simulink model "TRAS_LQI"  (R2021b)
settings: Solver=ode5  StartTime=0.0  StopTime=999  FixedStep=0.01  RelTol=1e-3  AbsTol=1e-6
values from neighbouring files (symbols this model uses):
  D = params.D    [x00_pendulum_identification.m]
  K = [9.60215440973 2.43688595265 0.00134146532326 3.16227766017]    [LQI_SETPOINT_CHANGE.mat]    (also in LQI_losowe_zaklocenie_i_maksymalne_zaklocenie_kilka_razy(ost_naj).mat; LQI_sam_z_ciezarem_znowu_sam.mat; LQR_losowe_zaklocenie_i_maksymalne_zaklocenie.mat = [8.82696664421 2.33839377811 0.00131075429192]; LQR_sam_z_ciezarem_znowu_sam.mat = [8.82696664421 2.33839377811 0.00131075429192])
  u_ref = u_ref_sol    [x03_pitch_control_model.m]
  x_ref = [theta_p_setpoint; 1e-12; omega_ref_sol]    [x03_pitch_control_model.m]
libraries: simulink x4, dspstat3 x3
settings Model: SimulationMode=external  ExtModeTrigDuration=12000  ExtModeTrigLevel=0.400000  Creator=jims  LastModifiedBy=STUDENT
settings SolverCC: AutoScaleAbsTol=off  AlgebraicLoopSolver=TrustRegion
settings DataIOCC: ExternalInput=[]  InitialState=[]  MaxDataPoints=5000  SaveFormat=Array  SignalLoggingSaveFormat=ModelDataLogs  SaveOutput=off  SaveTime=off  ReturnWorkspaceOutputs=off  SignalLoggingName=sigsOut
settings OptimizationCC: BooleanDataType=off  ExpressionDepthLimit=2147483647  InitFltsAndDblsToZero=on  LifeSpan=inf
settings DebuggingCC: SaveWithParameterizedLinksMsg=none  MultiTaskDSMMsg=warning  MultiTaskCondExecSysMsg=none  IntegerOverflowMsg=none  StateNameClashWarn=warning  SFUnexpectedBacktrackingDiag=warning  SFNoUnconditionalDefaultTransitionDiag=warning  SFExecutionAtInitializationDiag=none  SFMachineParentedDataDiag=warning  IntegerSaturationMsg=none  ArithmeticOperatorsInVariantConditions=warning
settings HardwareCC: TargetBitPerLong=64  TargetBitPerPointer=64  TargetIntDivRoundTo=Zero  TargetEndianess=LittleEndian  TargetWordSize=64  TargetHWDeviceType=Intel->x86-64
settings ModelReferenceCC: PropagateSignalLabelsOutOfModel=off
settings SFSimCC: SimUseLocalCustomCode=off  CustomCodeUndefinedFunction=UseInterfaceOnly
settings RTWCC: Description=Simulink Desktop Real-Time  SystemTargetFile=sldrt.tlc  TemplateMakefile=sldrt.tmf  RTWUseLocalCustomCode=off  RTWCompilerOptimization=on
settings CodeAppCC: MaxIdLength=95  StateflowObjectComments=on
settings SimulinkDesktopRealTimeCC: TargetFcnLib=ansi_tfl_tmw.mat  TargetPreCompLibLocation=C:\apps\MATLAB\R2021b\toolbox\sldrt\lib\win64  TargetLangStandard=C89/C90 (ANSI)  ModelReferenceCompliant=off  CompOptLevelCompliant=off  SupportVariableSizeSignals=off
settings ConfigComp: CovMetricSettings=dw  CovSaveCumulativeToWorkspaceVar=on  CovSaveSingleToWorkspaceVar=on  CovExternalEMLEnable=off

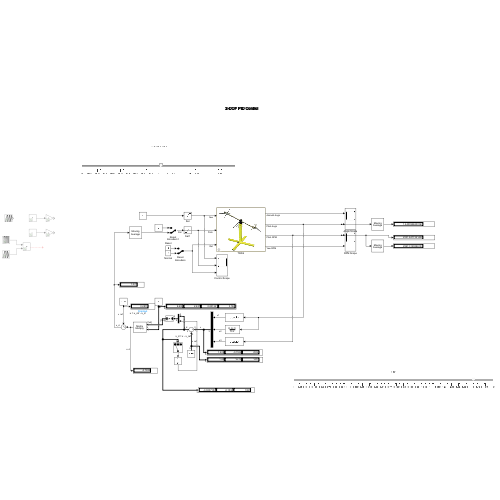
[thumbnail: Simulink's stored preview of the top-level diagram]
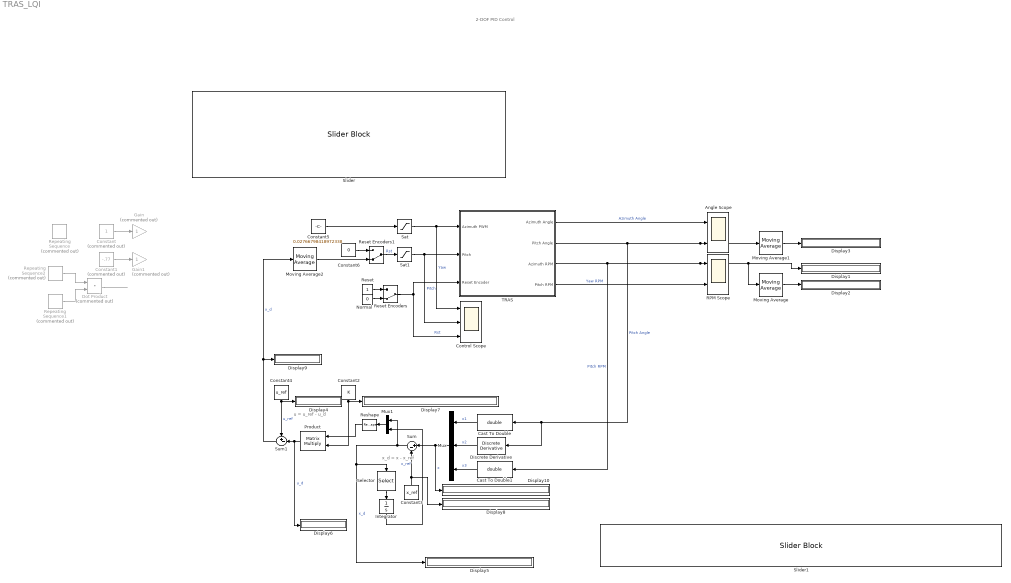
== system TRAS_LQI ==
  note: x_d = x - x_ref
  note: 2-DOF PID Control
  note: u = u_ref - u_d
  Angle Scope : Scope  NumInputPorts=2
  Cast To Double : DataTypeConversion  OutDataTypeStr=double
  Cast To Double1 : DataTypeConversion  OutDataTypeStr=double
  Constant : Constant  Commented=on
  Constant1 : Constant  Commented=on  Value=-.77
  Constant2 : Constant  Value=K
  Constant3 : Constant  Value=x_ref
  Constant4 : Constant  Value=u_ref
  Constant5 : Constant  Value=0.02766798418972338
  Constant6 : Constant  Value=0
  Control Scope : Scope  NumInputPorts=3
  Discrete Derivative : simulink/Discrete/Discrete Derivative  gainval=1.0  ICPrevScaledInput=0.0  OutMin=[]  OutMax=[]  OutDataType=fixdt(1, 16)  OutScaling=2^-10  DoSatur=off
  Display{1..10} (10 alike) : Display
  Dot Product : DotProduct  Commented=on  InputSameDT=on  OutDataTypeStr=Inherit: Inherit via internal rule
  Gain : Gain  Commented=on
  Gain1 : Gain  Commented=on
  Integrator : Integrator
  Moving Average : dspstat3/Moving Average  Method=Sliding window  ForgettingFactorPort=off  SpecifyWindowLength=on  WindowLength=100  ForgettingFactor=0.9  SimulateUsing=Code generation
  Moving Average1 : dspstat3/Moving Average  Method=Sliding window  ForgettingFactorPort=off  SpecifyWindowLength=on  WindowLength=100  ForgettingFactor=0.9  SimulateUsing=Code generation
  Moving Average2 : dspstat3/Moving Average  Method=Sliding window  ForgettingFactorPort=off  SpecifyWindowLength=on  WindowLength=10  ForgettingFactor=0.9  SimulateUsing=Code generation
  Mux : Mux  Inputs=3
  Mux1 : Mux  Inputs=2
  Normal : Constant  Value=0
  Product : Product  Multiplication=Matrix(*)
  RPM Scope : Scope  NumInputPorts=2
  Repeating Sequence : simulink/Sources/Repeating Sequence  Commented=on  rep_seq_t=[0 1 1.001 2 2.001 3 3.001 4 4.001 5 5.001 6 6.001 7 7.001 8 8.001 9 9.001 10 10.001 11]*10.  rep_seq_y=[0 0 1 1 2 2 3 3 4 4 5 5 6 6 7 7 8 8 9 9 10 10]/10
  Repeating Sequence1 : simulink/Sources/Repeating Sequence  Commented=on  rep_seq_t=[0 1 1.001 2 2.001 3 3.001 4 4.001 5 5.001 6 6.001 7 7.001 8 8.001 9 9.001 10 10.001 11]*20  rep_seq_y=[0 0 1 1 2 2 3 3 4 4 5 5 6 6 7 7 8 8 9 9 10 10]/10
  Repeating Sequence2 : simulink/Sources/Repeating Sequence  Commented=on  rep_seq_t=[0 10 10.001 20]  rep_seq_y=[0 0 1 1]
  Reset : Constant
  Reset Encoders : ManualSwitch  CurrentSetting=0
  Reset Encoders1 : ManualSwitch  CurrentSetting=0
  Reshape : Reshape  OutputDimensionality=Row vector (2-D)
  Sat : Saturate  UpperLimit=1  LowerLimit=-1
  Sat1 : Saturate  UpperLimit=1  LowerLimit=-1
  Selector : Selector  InputPortWidth=3  IndexOptions=Index vector (dialog)  Indices=[1]  OutputSizes=1
  Slider : SliderBlock  ScaleMin=-1  ScaleMax=1
  Slider1 : SliderBlock  ScaleMax=1.6
  Sum : Sum  Inputs=|+-
  Sum1 : Sum  Inputs=+-|
  TRAS : Subsystem  mask{BaseAddress=57088, T0=0.01}
      mask prompts: BaseAddress "Base Address:"; T0 "Sampling Period:"
      mask Display: image('TRAS.JPG')
  wires:
  Sat/1 -> TRAS/1(Azimuth PWM), Control Scope/1  "Yaw"
  Sat1/1 -> Control Scope/2, TRAS/2(Pitch)  "Pitch"
  Reset Encoders/1 -> TRAS/3(Reset Encoder), Control Scope/3  "Rst"
  Reset/1 -> Reset Encoders/1
  Normal/1 -> Reset Encoders/2
  TRAS/4(Pitch RPM) -> RPM Scope/2  "Yaw RPM"
  TRAS/3(Azimuth RPM) -> Cast To Double1/1, Display1/1, Moving Average/1, RPM Scope/1  "Pitch RPM"
  TRAS/1(Azimuth Angle) -> Angle Scope/1  "Azimuth Angle"
  TRAS/2(Pitch Angle) -> Discrete Derivative/1, Cast To Double/1, Moving Average1/1, Angle Scope/2  "Pitch Angle"
  Moving Average/1 -> Display2/1
  Moving Average1/1 -> Display3/1
  Repeating Sequence2/1 -> Dot Product/1
  Repeating Sequence1/1 -> Dot Product/2
  Constant1/1 -> Gain1/1
  Dot Product/1 -> ?
  Constant/1 -> Gain/1
  Cast To Double/1 -> Mux/1  "x1"
  Cast To Double1/1 -> Mux/3  "x3"
  Discrete Derivative/1 -> Mux/2  "x2"
  Mux/1 -> Display10/1, Sum/1  "x"
  Constant3/1 -> Display8/1, Sum/2  "x_ref"
  Sum/1 -> Selector/1, Display5/1, Mux1/1  "x_d"
  Product/1 -> Display6/1, Sum1/2  "u_d"
  Constant4/1 -> Display4/1, Sum1/1  "u_ref"
  Sum1/1 -> Display9/1, Moving Average2/1  "x_d"
  Constant2/1 -> Product/2, Display7/1
  Reset Encoders1/1 -> Sat1/1  "Rst"
  Constant6/1 -> Reset Encoders1/1
  Moving Average2/1 -> Reset Encoders1/2
  Selector/1 -> Integrator/1
  Integrator/1 -> Mux1/2
  Mux1/1 -> Reshape/1
  Reshape/1 -> Product/1
  Constant5/1 -> Sat/1

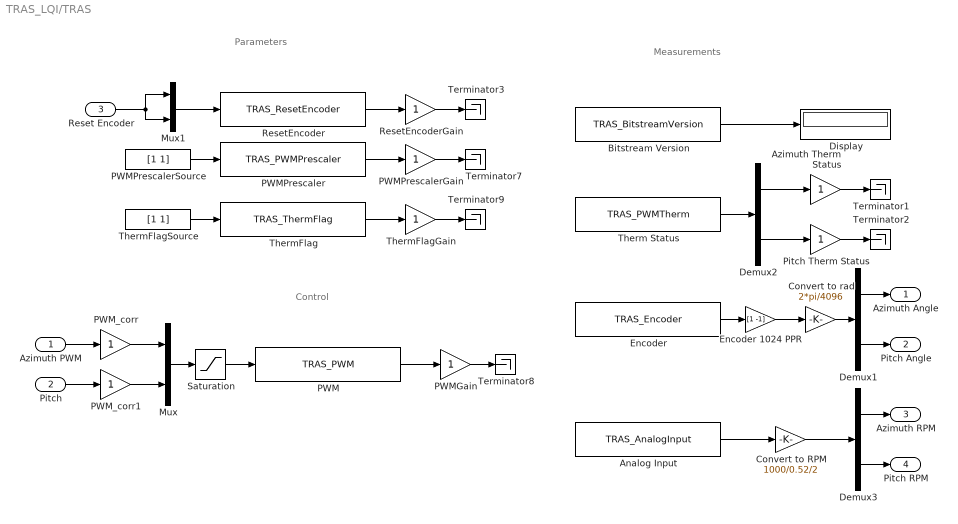
== system TRAS_LQI/TRAS ==
  note: Parameters
  note: Control
  note: Measurements
  Azimuth PWM : Inport
  Pitch : Inport  Port=2
  Reset Encoder : Inport  Port=3
  Analog Input : S-Function  FunctionName=TRAS_AnalogInput  Parameters=BaseAddress, [1 0], [1 1], T0  SFunctionDeploymentMode=off  EnableBusSupport=off
  Azimuth Therm Status : Gain  SaturateOnIntegerOverflow=on  OutDataTypeStr=Inherit: Same as input  ParamDataTypeStr=Inherit: Same as input
  Bitstream Version : S-Function  FunctionName=TRAS_BitstreamVersion  Parameters=BaseAddress, T0  SFunctionDeploymentMode=off  EnableBusSupport=off
  Convert to RPM : Gain  Gain=1000/0.52/2  SaturateOnIntegerOverflow=on  OutDataTypeStr=Inherit: Same as input  ParamDataTypeStr=Inherit: Same as input
  Convert to rad : Gain  Gain=2*pi/4096  SaturateOnIntegerOverflow=on  OutDataTypeStr=Inherit: Same as input  ParamDataTypeStr=Inherit: Same as input
  Demux1 : Demux  Outputs=2
      settings: DisplayOption=none
  Demux2 : Demux  Outputs=2
      settings: DisplayOption=none
  Demux3 : Demux  Outputs=2
      settings: DisplayOption=none
  Display : Display
  Encoder : S-Function  FunctionName=TRAS_Encoder  Parameters=BaseAddress, T0  SFunctionDeploymentMode=off  EnableBusSupport=off
  Encoder 1024 PPR : Gain  Gain=[1 -1]  SaturateOnIntegerOverflow=on  OutDataTypeStr=Inherit: Same as input  ParamDataTypeStr=Inherit: Same as input
  Mux : Mux  Inputs=2
  Mux1 : Mux  Inputs=2
  PWM : S-Function  FunctionName=TRAS_PWM  Parameters=BaseAddress, T0  SFunctionDeploymentMode=off  EnableBusSupport=off
  PWMGain : Gain  SaturateOnIntegerOverflow=on  OutDataTypeStr=Inherit: Same as input  ParamDataTypeStr=Inherit: Same as input
  PWMPrescaler : S-Function  FunctionName=TRAS_PWMPrescaler  Parameters=BaseAddress, T0  SFunctionDeploymentMode=off  EnableBusSupport=off
  PWMPrescalerGain : Gain  SaturateOnIntegerOverflow=on  OutDataTypeStr=Inherit: Same as input  ParamDataTypeStr=Inherit: Same as input
  PWMPrescalerSource : Constant  Value=[1 1]
  PWM_corr : Gain  SaturateOnIntegerOverflow=on  OutDataTypeStr=Inherit: Same as input  ParamDataTypeStr=Inherit: Same as input
  PWM_corr1 : Gain  SaturateOnIntegerOverflow=on  OutDataTypeStr=Inherit: Same as input  ParamDataTypeStr=Inherit: Same as input
  Pitch Therm Status : Gain  SaturateOnIntegerOverflow=on  OutDataTypeStr=Inherit: Same as input  ParamDataTypeStr=Inherit: Same as input
  ResetEncoder : S-Function  FunctionName=TRAS_ResetEncoder  Parameters=BaseAddress, T0  SFunctionDeploymentMode=off  EnableBusSupport=off
  ResetEncoderGain : Gain  SaturateOnIntegerOverflow=on  OutDataTypeStr=Inherit: Same as input  ParamDataTypeStr=Inherit: Same as input
  Saturation : Saturate  UpperLimit=1  LowerLimit=-1
  Terminator{1..3,7..9} (6 alike) : Terminator
  Therm Status : S-Function  FunctionName=TRAS_PWMTherm  Parameters=BaseAddress, T0  SFunctionDeploymentMode=off  EnableBusSupport=off
  "ThermFlag " : S-Function  FunctionName=TRAS_ThermFlag  Parameters=BaseAddress, T0  SFunctionDeploymentMode=off  EnableBusSupport=off
  ThermFlagGain : Gain  SaturateOnIntegerOverflow=on  OutDataTypeStr=Inherit: Same as input  ParamDataTypeStr=Inherit: Same as input
  ThermFlagSource : Constant  Value=[1 1]
  Azimuth Angle : Outport
  Pitch Angle : Outport  Port=2
  Azimuth RPM : Outport  Port=3
  Pitch RPM : Outport  Port=4
  wires:
  Encoder 1024 PPR/1 -> Convert to rad/1
  Encoder/1 -> Encoder 1024 PPR/1
  Saturation/1 -> PWM/1
  Mux/1 -> Saturation/1
  PWM/1 -> PWMGain/1
  PWMGain/1 -> Terminator8/1
  ResetEncoder/1 -> ResetEncoderGain/1
  PWMPrescaler/1 -> PWMPrescalerGain/1
  Mux1/1 -> ResetEncoder/1
  PWMPrescalerSource/1 -> PWMPrescaler/1
  ResetEncoderGain/1 -> Terminator3/1
  PWMPrescalerGain/1 -> Terminator7/1
  Demux1/2 -> Pitch Angle/1
  Convert to rad/1 -> Demux1/1
  Demux1/1 -> Azimuth Angle/1
  Therm Status/1 -> Demux2/1
  Demux2/2 -> Pitch Therm Status/1
  Demux2/1 -> Azimuth Therm Status/1
  Azimuth Therm Status/1 -> Terminator1/1
  Pitch Therm Status/1 -> Terminator2/1
  Bitstream Version/1 -> Display/1
  Analog Input/1 -> Convert to RPM/1
  Demux3/2 -> Pitch RPM/1
  Demux3/1 -> Azimuth RPM/1
  Reset Encoder/1 -> Mux1/1, Mux1/2
  Convert to RPM/1 -> Demux3/1
  "ThermFlag "/1 -> ThermFlagGain/1
  ThermFlagSource/1 -> "ThermFlag "/1
  ThermFlagGain/1 -> Terminator9/1
  Azimuth PWM/1 -> PWM_corr/1
  PWM_corr/1 -> Mux/1
  Pitch/1 -> PWM_corr1/1
  PWM_corr1/1 -> Mux/2
